simulink model "d3_model_AdaptiveAudio"  (R2020a)
settings: Solver=ode45  StartTime=0.0  StopTime=20  RelTol=1e-3  EnableMultiTasking=on
libraries: dspsnks4 x2, dspvision x2, dspadpt3 x1
settings Model: ModifiedByFormat=The MathWorks Inc.  Creator=The MathWorks, Inc.  LastModifiedBy=The MathWorks Inc.
settings DataIOCC: LimitDataPoints=on  SaveFormat=Array  ReturnWorkspaceOutputs=off  SignalLoggingName=logsOut
settings OptimizationCC: ExpressionDepthLimit=2147483647  InitFltsAndDblsToZero=on  EfficientMapNaN2IntZero=off  LifeSpan=inf
settings DebuggingCC: UnderspecifiedInitializationDetection=Classic  MergeDetectMultiDrivingBlocksExec=none  SignalResolutionControl=TryResolveAllWithWarning  MultiTaskDSMMsg=warning  MultiTaskCondExecSysMsg=none  ParameterPrecisionLossMsg=none  FcnCallInpInsideContextMsg=warning  StateNameClashWarn=warning  SFUnexpectedBacktrackingDiag=warning  SFNoUnconditionalDefaultTransitionDiag=warning  SFExecutionAtInitializationDiag=none  ArithmeticOperatorsInVariantConditions=warning
settings HardwareCC: ProdBitPerPointer=32  ProdBitPerSizeT=32  ProdBitPerPtrDiffT=32  ProdLargestAtomicFloat=None  ProdIntDivRoundTo=Undefined  ProdEndianess=Unspecified  ProdWordSize=32  ProdHWDeviceType=Specified
settings ModelReferenceCC: PropagateSignalLabelsOutOfModel=off
settings SFSimCC: SimUseLocalCustomCode=off  CustomCodeUndefinedFunction=UseInterfaceOnly
settings RTWCC: RTWUseLocalCustomCode=off
settings CodeAppCC: StateflowObjectComments=on
settings GRTTargetCC: TargetFcnLib=ansi_tfl_tmw_new.mat  TargetLangStandard=C89/C90 (ANSI)  CombineOutputUpdateFcns=off  GRTInterface=on
settings ConfigComp: CovMetricSettings=dw  CovHtmlReporting=on  CovSaveCumulativeToWorkspaceVar=on  CovSaveSingleToWorkspaceVar=on  CovExternalEMLEnable=off  CovSFcnEnable=off

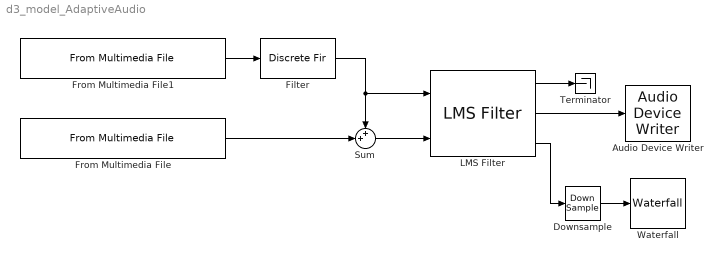
== system d3_model_AdaptiveAudio ==
  Audio Device Writer : dspsnks4/Audio Device Writer  Driver=DirectSound  Device=Default  InheritSampleRate=on  SampleRate=44100  BitDepth=16-bit integer  BufferSize=4096  NumBuffers=10  DefaultOutputChannelMapping=on  OutputChannelMapping=1:2  OutputNumUnderrunSamples=off  DriverIdx=1  DeviceWarnFlag=''
  Downsample : DownSample  N=32  RateOptions=Allow multirate processing
  Filter : DiscreteFir  Tag=BlockMethodSubSystem  Coefficients=[-7.31261440035516682e-05 -9.31955213052300944e-05 -3.06044825197509959e-05 0.000164179418333110396 0.000416447028969218211 0.000517314220350287984 0.000228928280019854242 -0.000504581007832899625 -0.00137399283301260712 -0.00173741793869143534 -0.000966385776089857145 0.0010200443535864506 0.00338282318454040647 0.00453954447297958384 0.00301318160864911134 -0.00140052295368660882 -0.00689683388783525995 -0.0100880331112129067 -0.00774970575771750068 0.000849663230186380007 0.0124481569612788553 0.0204436399397609145 0.0180091300712826273 0.0024635753411626762 -0.0214513470186862981 -0.0416836047737839943 -0.0431890885239163275 -0.0149988912124264257 0.0432597516233297272 0.118933961704835001 0.189853668835169243 0.232720688346417903 0.232720688346417903 0.189853668835169243 0.118933961704835001 0.0432597516233297272 -0.0149988912124264257 -0.0431890885239163275 -0.0416836047737839943 -0.0214513470186862981 0.0024635753411626762 0.0180091300712826273 0.0204436399397609145 0.0124481569612788553 0.000849663230186380007 -0.00774970575771750068 -0.0100880331112129067 -0.00689683388783525995 -0.00140052295368660882 0.00301318160864911134 0.00453954447297958384 0.00338282318454040647 0.0010200443535864506 -0.000966385776089857145 -0.00173741793869143534 -0.00137399283301260712 -0.000504581007832899625 0.000228928280019854242 0.000517314220350287984 0.000416447028969218211 0.000164179418333110396 -3.06044825197509959e-05 -9.31955213052300944e-05 -7.31261440035516682e-05]  InputProcessing=Columns as channels (frame based)
  From Multimedia File : dspvision/From Multimedia File  inputFilename=debussy.mp3  readRange=[1 Inf]  loop=on  numPlays=inf  outputStreams=Audio only  videoDataType=single  audioDataType=double  inheritSampleTime=on  userDefinedSampleTime=1/30  noAudioOutput=off  isIntensityVideo=off  fourcc=RGB  colorVideoFormat=Separate color signals  outputEOF=off  dataOrg=Column-major  audioFrameSize=100  computeAudioFrameSize=off  outSamplingMode=Sample based
  From Multimedia File1 : dspvision/From Multimedia File  inputFilename=whistle.mp3  readRange=[1 Inf]  loop=on  numPlays=inf  outputStreams=Audio only  videoDataType=single  audioDataType=double  inheritSampleTime=on  userDefinedSampleTime=1/30  noAudioOutput=off  isIntensityVideo=off  fourcc=RGB  colorVideoFormat=Separate color signals  outputEOF=off  dataOrg=Column-major  audioFrameSize=100  computeAudioFrameSize=off  outSamplingMode=Sample based
  LMS Filter : dspadpt3/LMS Filter  Algo=LMS  L=64  stepflag=Dialog  mu=0.0005  leakage=1  ic=0  Adapt=off  resetflag=None  weights=on  addnparflag=off  roundingMode=Floor  overflowMode=off  secondCoeffMode=Binary point scaling  secondCoeffWordLength=2  secondCoeffFracLength=15  prodOutput2Mode=Binary point scaling  prodOutput2FracLength=20  prodOutput3Mode=Binary point scaling  prodOutput3FracLength=20  prodOutput4Mode=Binary point scaling  prodOutput4FracLength=20  quotientMode=Binary point scaling  quotientFracLength=20  accum2Mode=Binary point scaling  accum2FracLength=20
      settings: SourceProductBaseCode=DS
  Sum : Sum  Inputs=++|
  Terminator : Terminator
  Waterfall : dspsnks4/Waterfall  TraceProperties=off  NumTraces=6  CMapStr=autumn  TNewest=1  TOldest=0  HistoryLength=50  HistoryFull=Overwrite  UpdateInterval=1  ExportMode=All visible  MLExportName=ExportData  AutoExport=off  DisplayProperties=off  MouseMode=Orbit  AxisGrid=on  Snapshot=off  Suspend=off  SyncSnapshots=off  OpenScopeAtSimStart=off  FigPos=[243 195 405 320]  CameraView=[69.4600750684385 564.426060114276 -133.474523953492 0 18.5 3.5 0.616338299486424 -7.9078811427274 1.98411164834144 0.461072183866044 1 196.185286103542 16.3487738419619]  InportDimsHint=[64 1]  AxisProperties=off  AxisColor='w'  XLabel=Amplitude  YLabel=Samples  ZLabel=Time  TriggerProperties=off  TrigStartMode=Immediately  TrigStartT=0  TrigStartN=0  TrigStartFcn=trigbegin  TrigStopMode=Never  TrigStopT=0.1  TrigStopN=1  TrigStopFcn=trigend  TrigRearmMode=Never  TrigRearmT=0  TrigRearmN=0  TrigRearmFcn=trigrearm  XformProperties=on  XformMode=None  XformFcn=abs  XformExpr=(u+1)/2
      settings: SourceProductBaseCode=DS  YMin=-0.188  YMax=0.179
  wires:
  From Multimedia File1/1 -> Filter/1
  LMS Filter/1 -> Terminator/1
  LMS Filter/2 -> Audio Device Writer/1
  LMS Filter/3 -> Downsample/1
  Downsample/1 -> Waterfall/1
  Sum/1 -> LMS Filter/2
  From Multimedia File/1 -> Sum/2
  Filter/1 -> LMS Filter/1, Sum/1
